simulink model "comparesansetavec"  (R2017a)
settings: Solver=VariableStepAuto  StartTime=0.0  StopTime=30  RelTol=1e-3
settings Model: Creator=pc  LastModifiedBy=pc

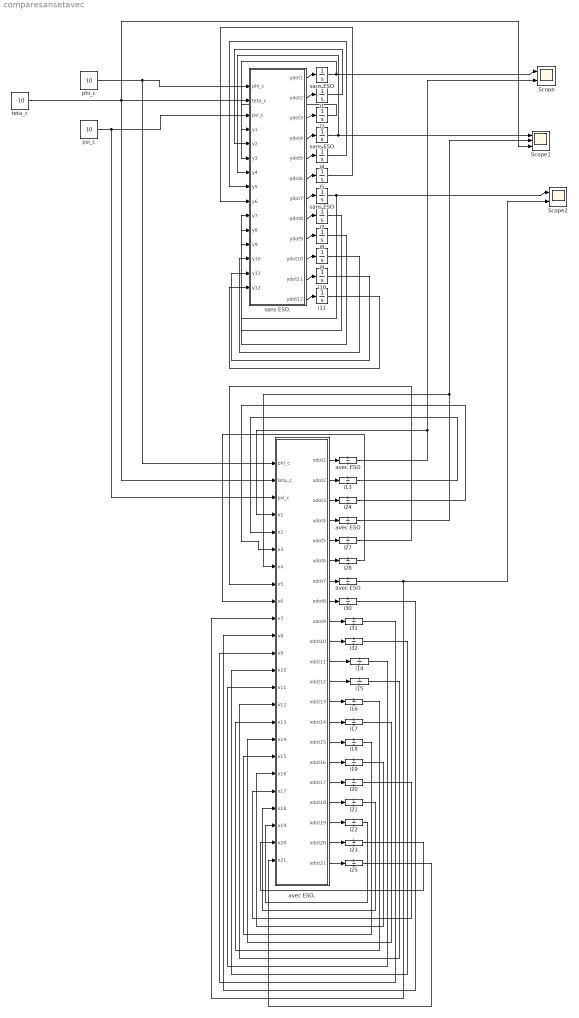
== system comparesansetavec ==
  Scope : Scope  NumInputPorts=2
  Scope1 : Scope  NumInputPorts=3
  Scope2 : Scope  NumInputPorts=2
  avec ESO : Integrator
  "avec ESO " : Integrator
  "avec ESO  " : Integrator
  avec ESO. : MATLAB Function  TreatAsAtomicUnit=on
  i{1..2,4..5,7..11,13..25,27..28,30..32} (27 alike) : Integrator
  phi_c : Constant  Value=10
  psi_c : Constant  Value=10
  sans ESO : Integrator
  "sans ESO " : Integrator
  "sans ESO  " : Integrator
  sans ESO. : MATLAB Function  TreatAsAtomicUnit=on
  teta_c : Constant  Value=-10
  wires:
  i10/1 -> sans ESO./14(y11)
  i5/1 -> sans ESO./9(y6)
  i7/1 -> sans ESO./11(y8)
  i1/1 -> sans ESO./5(y2)
  sans ESO./7(ydot7) -> "sans ESO "/1
  i2/1 -> sans ESO./6(y3)
  "sans ESO "/1 -> Scope2/1, sans ESO./10(y7)
  "sans ESO  "/1 -> Scope/1, sans ESO./4(y1)
  sans ESO./10(ydot10) -> i9/1
  sans ESO./4(ydot4) -> sans ESO/1
  sans ESO./3(ydot3) -> i2/1
  sans ESO/1 -> Scope1/1, sans ESO./7(y4)
  i4/1 -> sans ESO./8(y5)
  sans ESO./2(ydot2) -> i1/1
  sans ESO./9(ydot9) -> i8/1
  i11/1 -> sans ESO./15(y12)
  sans ESO./12(ydot12) -> i11/1
  sans ESO./1(ydot1) -> "sans ESO  "/1
  sans ESO./8(ydot8) -> i7/1
  sans ESO./11(ydot11) -> i10/1
  i8/1 -> sans ESO./12(y9)
  sans ESO./6(ydot6) -> i5/1
  i9/1 -> sans ESO./13(y10)
  sans ESO./5(ydot5) -> i4/1
  avec ESO./6(xdot6) -> i28/1
  i28/1 -> avec ESO./9(x6)
  i13/1 -> avec ESO./5(x2)
  avec ESO./14(xdot14) -> i17/1
  i17/1 -> avec ESO./17(x14)
  avec ESO./13(xdot13) -> i16/1
  avec ESO./2(xdot2) -> i13/1
  i22/1 -> avec ESO./22(x19)
  avec ESO./5(xdot5) -> i27/1
  avec ESO./9(xdot9) -> i31/1
  i25/1 -> avec ESO./24(x21)
  i21/1 -> avec ESO./21(x18)
  i20/1 -> avec ESO./20(x17)
  avec ESO./3(xdot3) -> i24/1
  avec ESO./12(xdot12) -> i15/1
  i15/1 -> avec ESO./15(x12)
  avec ESO./4(xdot4) -> avec ESO/1
  "avec ESO  "/1 -> Scope/2, avec ESO./4(x1)
  i23/1 -> avec ESO./23(x20)
  avec ESO/1 -> Scope1/2, avec ESO./7(x4)
  phi_c/1 -> avec ESO./1(phi_c), sans ESO./1(phi_c)
  i24/1 -> avec ESO./6(x3)
  i16/1 -> avec ESO./16(x13)
  "avec ESO "/1 -> avec ESO./10(x7), Scope2/2
  psi_c/1 -> avec ESO./3(psi_c), sans ESO./3(psi_c)
  i30/1 -> avec ESO./11(x8)
  i18/1 -> avec ESO./18(x15)
  teta_c/1 -> avec ESO./2(teta_c), Scope1/3, sans ESO./2(teta_c)
  avec ESO./18(xdot18) -> i21/1
  i27/1 -> avec ESO./8(x5)
  i31/1 -> avec ESO./12(x9)
  avec ESO./8(xdot8) -> i30/1
  avec ESO./1(xdot1) -> "avec ESO  "/1
  avec ESO./10(xdot10) -> i32/1
  avec ESO./16(xdot16) -> i19/1
  avec ESO./15(xdot15) -> i18/1
  avec ESO./21(xdot21) -> i25/1
  avec ESO./19(xdot19) -> i22/1
  avec ESO./7(xdot7) -> "avec ESO "/1
  avec ESO./20(xdot20) -> i23/1
  i19/1 -> avec ESO./19(x16)
  i14/1 -> avec ESO./14(x11)
  avec ESO./11(xdot11) -> i14/1
  i32/1 -> avec ESO./13(x10)
  avec ESO./17(xdot17) -> i20/1

== matlab function comparesansetavec/avec ESO. ==
  data: phi_c input; teta_c input; psi_c input; xdot1 output; x1 input; x2 input; x3 input; x4 input; x5 input; x6 input; x7 input; x8 input; x9 input; x10 input; x11 input; x12 input; x13 input; x14 input; x15 input; x16 input; x17 input; x18 input; x19 input; x20 input; x21 input; xdot2 output; xdot3 output; xdot4 output; xdot5 output; xdot6 output; xdot7 output; xdot8 output; xdot9 output; xdot10 output; xdot11 output; xdot12 output; xdot13 output; xdot14 output; xdot15 output; xdot16 output; xdot17 output; xdot18 output; xdot19 output; xdot20 output; xdot21 output
function [xdot1,xdot2,xdot3,xdot4,xdot5,xdot6,xdot7,xdot8,xdot9,xdot10,xdot11,xdot12,xdot13,xdot14,xdot15,xdot16,xdot17,xdot18,xdot19,xdot20,xdot21] = fcn(phi_c,teta_c,psi_c,x1,x2,x3,x4,x5,x6,x7,x8,x9,x10,x11,x12,x13,x14,x15,x16,x17,x18,x19,x20,x21)
alfa1=0.9; alfa2=0.3;
delta=0.1;
kd1=6.4;kd2=6.4;kd3=6.4;
kp1=16;kp2=16;kp3=16;
beta1=100; beta2=3000; beta3=5000;
%--------------------------------------------------------------------------
Ix=22682;
Iy=77095;
Iz=95561;
Ixz=1125;
SOM=Ix*Iz-Ixz^2;
c1=((Iy-Iz)*Iz-Ixz^2)/SOM;
c2=((Ix-Iy+Iz)*Ixz)/SOM;
c3=Iz/SOM;
c4=Ixz/SOM;
c5=(Iz-Ix)/Iy;
c6=Ixz/Iy;
c7=1/Iy;
c8=(Ix*(Ix-Iy)+Ixz^2)/SOM;
c9=Ix/SOM;
%--------------------------------------------------------------------------
phi=x1;
teta=x4;
p=x19;
r=x20;
q=x21;
%--------------------------------------------------------------------------
B=[c3+c4*cosd(phi)*tand(teta),c7*sind(phi)*tand(teta),c4+c9*cosd(phi)*tand(teta);
    -c4*sind(phi),c7*cosd(phi),-c9*sind(phi);
    c4*cosd(phi)*(1/cosd(teta)),c7*sind(phi)*(1/cosd(teta)),c9*cosd(phi)*(1/cosd(teta))];
phidot=p+tand(teta)*(q*sind(phi)+r*cosd(phi));
tetadot=q*cosd(phi)-r*sind(phi);
A1=((c1*r+c2*p)*q)+(tetadot/cosd(teta)^2)*(q*sind(phi)+r*cosd(phi))+tand(teta)*((c5*p*r-c6*(p^2-r^2))*sind(phi)+q*(phidot*cosd(phi))+((c8*p-c2*r)*q)*cosd(phi)-r*phidot*sind(phi));
A2=(c5*p*r-c6*(p^2-r^2))*cosd(phi)-phidot*sind(phi)*q-(((c8*p-c2*r)*q)*sind(phi)+phidot*cosd(phi)*r);
A3=((c5*p*r-c6*(p^2-r^2))*sind(phi)+phidot*cosd(phi)*q+((c8*p-c2*r)*q)*cosd(phi)-phidot*sind(phi)*r)*cosd(teta)/cosd(teta)^2+(tetadot*sind(teta)*(q*sind(phi)+r*cosd(phi)))/cosd(teta)^2;
%--------------------------------------------------------------------------
pp=inv(B);
L=pp(1,:)*[(kp1*phi_c-x12)-A1;(kp2*teta_c-x15)-A2;(kp3*psi_c-x18)-A3];
M=pp(2,:)*[(kp1*phi_c-x12)-A1;(kp2*teta_c-x15)-A2;(kp3*psi_c-x18)-A3];
N=pp(3,:)*[(kp1*phi_c-x12)-A1;(kp2*teta_c-x15)-A2;(kp3*psi_c-x18)-A3];
%************------************----------**************-----------------
e=x10-x1;                                     %y(1)=phi y(10)=Z1_phi 
e2=x13-x4;                                      %y(4)=teta y(14)=Z1_teta
e3=x16-x7;                                      %y(7)=psi y(16)=Z1_PSI
%************------************----------**************-----------------
xdot1=x2;   
%xdot2=A1+B(1,:)*[L;M;N];
xdot2=x3+kp1*phi_c;
%xdot3=A1dot+Bdot(1,:)*u+B(1,:)*udot;
Delta_u1=x12+kp1*x1+kd1*x2;
xdot3=-kp1*x2-kd1*(x3+kp1*phi_c)-Delta_u1;
%---ESO1 Z_PHI---
xdot10=x11-beta1*e;                           %y(11)=Z2_phi
%^^^^^^^^^^^^^^^^^^^^^^^^^^^^^^^^^^^^^^^^^^^^^^^^^^^^^^^^^^^^^^^^^^^^^^^^^^
if abs(e)> delta 
FAL=abs(e)^alfa1*sign(e);
xdot11=x12-beta2*FAL+kp1*phi_c;%y(12)=Z3_phi
else 
    FAL=e/(delta^(1-alfa1));
 xdot11=x12-beta2*FAL+kp1*phi_c;%y(12)=Z3_phi
end
%^^^^^^^^^^^^^^^^^^^^^^^^^^^^^^^^^^^^^^^^^^^^^^^^^^^^^^^^^^^^^^^^^^^^^^^^^^ 
if abs(e)> delta 
FAL1=abs(e)^alfa2*sign(e);
xdot12=-beta3*FAL1;
else 
    FAL1=e/(delta^(1-alfa2));
    xdot12=-beta3*FAL1;
end
%^^^^^^^^^^^^^^^^^^^^^^^^^^^^^^^^^^^^^^^^^^^^^^^^^^^^^^^^^^^^^^^^^^^^^^^^^^


%--------------------------------------------------------------------------
xdot4=x5;   
%xdot4=A2+B(2,:)*[L;M;N];  
xdot5=x6+kp2*teta_c;
%xdot6=A2dot+Bdot(2,:)*u+B(2,:)*udot;
Delta_u2=x15+kp2*x4+kd2*x5;
xdot6=-kp2*x5-kd1*(x6+kp2*teta_c)-Delta_u2;
%---ESO2 Z_Teta---
xdot13=x14-beta1*e2;                            %y(15)=Z2_teta
%^^^^^^^^^^^^^^^^^^^^^^^^^^^^^^^^^^^^^^^^^^^^^^^^^^^^^^^^^^^^^^^^^^^^^^^^^^
if abs(e2)> delta 
FAL2=abs(e2)^alfa1*sign(e2);
xdot14=x15-beta2*FAL2+kp2*teta_c;%y(16)=Z3_teta 
else
    FAL2=e2/(delta^(1-alfa1));
xdot14=x15-beta2*FAL2+kp2*teta_c;%y(16)=Z3_teta 
end
%^^^^^^^^^^^^^^^^^^^^^^^^^^^^^^^^^^^^^^^^^^^^^^^^^^^^^^^^^^^^^^^^^^^^^^^^^^ 
if abs(e2)> delta 
FAL3=abs(e2)^alfa2*sign(e2);
xdot15=-beta3*FAL3;
else
    FAL3=e2/(delta^(1-alfa2));
xdot15=-beta3*FAL3;
end
%^^^^^^^^^^^^^^^^^^^^^^^^^^^^^^^^^^^^^^^^^^^^^^^^^^^^^^^^^^^^^^^^^^^^^^^^^^


%--------------------------------------------------------------------------
xdot7=x8;   
%xdot6=A3+B(3,:)*[L;M;N];
xdot8=x9+kp3*psi_c;
%xdot9=A3dot+Bdot(3,:)*u+B(3,:)*udot;
Delta_u3=x18+kp3*x7+kd3*x8;
xdot9=-kp3*x8-kd3*(x9+kp3*psi_c)-Delta_u3;
%---ESO3 Z_PSI---
xdot16=x17-beta1*e3;                          %y(17)=Z2_PSI
%^^^^^^^^^^^^^^^^^^^^^^^^^^^^^^^^^^^^^^^^^^^^^^^^^^^^^^^^^^^^^^^^^^^^^^^^^^
if abs(e3)> delta 
FAL4=abs(e3)^alfa1*sign(e3);
xdot17=x18-beta2*FAL4+kp3*psi_c; %y(18)=Z3_PSI
else
    FAL4=e3/(delta^(1-alfa1));
xdot17=x18-beta2*FAL4+kp3*psi_c; %y(18)=Z3_PSI
end
%^^^^^^^^^^^^^^^^^^^^^^^^^^^^^^^^^^^^^^^^^^^^^^^^^^^^^^^^^^^^^^^^^^^^^^^^^^ 
if abs(e3)> delta 
FAL5=abs(e3)^alfa2*sign(e3);
xdot18=-beta3*FAL5;
else
    FAL5=e3/(delta^(1-alfa2));
xdot18=-beta3*FAL5;
end
%^^^^^^^^^^^^^^^^^^^^^^^^^^^^^^^^^^^^^^^^^^^^^^^^^^^^^^^^^^^^^^^^^^^^^^^^^^

%--------------------------------------------------------------------------
xdot19=(c1*r+c2*p)*q+c3*L+c4*N;  %=pdot
xdot20=(c8*p-c2*r)*q+c4*L+c9*N;  %=rdot
xdot21=c5*p*r-c6*(p^2-r^2)+c7*M; %=qdot
end

== matlab function comparesansetavec/sans ESO. ==
  data: phi_c input; teta_c input; psi_c input; y1 input; ydot1 output; y2 input; y3 input; y4 input; y5 input; y6 input; y7 input; y8 input; y9 input; y10 input; y11 input; y12 input; ydot2 output; ydot3 output; ydot4 output; ydot5 output; ydot6 output; ydot7 output; ydot8 output; ydot9 output; ydot10 output; ydot11 output; ydot12 output
function [ydot1,ydot2,ydot3,ydot4,ydot5,ydot6,ydot7,ydot8,ydot9,ydot10,ydot11,ydot12] = fcn(phi_c,teta_c,psi_c,y1,y2,y3,y4,y5,y6,y7,y8,y9,y10,y11,y12)
kd1=6.4;kd2=6.4;kd3=6.4;
kp1=16;kp2=16;kp3=16;
%--------------------------------------------------------------------------
% Ix=12874.8;
% Iy=75673.6;
% Iz=85552.1;
% Ixz=1331.4;
Ix=22682;
Iy=77095;
Iz=95561;
Ixz=1125;
SOM=Ix*Iz-Ixz^2;
c1=((Iy-Iz)*Iz-Ixz^2)/SOM;
c2=((Ix-Iy+Iz)*Ixz)/SOM;
c3=Iz/SOM;
c4=Ixz/SOM;
c5=(Iz-Ix)/Iy;
c6=Ixz/Iy;
c7=1/Iy;
c8=(Ix*(Ix-Iy)+Ixz^2)/SOM;
c9=Ix/SOM;
%--------------------------------------------------------------------------
phi=y1;
teta=y4;
p=y10;
r=y11;
q=y12;
%--------------------------------------------------------------------------
B=[c3+c4*cosd(phi)*tand(teta),c7*sind(phi)*tand(teta),c4+c9*cosd(phi)*tand(teta);
    -c4*sind(phi),c7*cosd(phi),-c9*sind(phi);
    c4*cosd(phi)*(1/cosd(teta)),c7*sind(phi)*(1/cosd(teta)),c9*cosd(phi)*(1/cosd(teta))];
phidot=p+tand(teta)*(q*sind(phi)+r*cosd(phi));
tetadot=q*cosd(phi)-r*sind(phi);
A1=((c1*r+c2*p)*q)+(tetadot/cosd(teta)^2)*(q*sind(phi)+r*cosd(phi))+tand(teta)*((c5*p*r-c6*(p^2-r^2))*sind(phi)+q*(phidot*cosd(phi))+((c8*p-c2*r)*q)*cosd(phi)-r*phidot*sind(phi));
A2=(c5*p*r-c6*(p^2-r^2))*cosd(phi)-phidot*sind(phi)*q-(((c8*p-c2*r)*q)*sind(phi)+phidot*cosd(phi)*r);
A3=((c5*p*r-c6*(p^2-r^2))*sind(phi)+phidot*cosd(phi)*q+((c8*p-c2*r)*q)*cosd(phi)-phidot*sind(phi)*r)*cosd(teta)/cosd(teta)^2+(tetadot*sind(teta)*(q*sind(phi)+r*cosd(phi)))/cosd(teta)^2;
A=[A1;A2;A3];
%--------------------------------------------------------------------------
Bdot=[c4*cosd(phi)*(tand(teta)^2 + 1)*tetadot - c4*sind(phi)*tand(teta)*phidot,c7*cosd(phi)*tand(teta)*phidot + c7*sind(phi)*(tand(teta)^2 + 1)*tetadot,c9*cosd(phi)*(tand(teta)^2 + 1)*tetadot - c9*sind(phi)*tand(teta)*phidot;
     -c4*cosd(phi)*phidot,-c7*sind(phi)*phidot,-c9*cosd(phi)*phidot;
     (c4*cosd(phi)*sind(teta)*tetadot)/cosd(teta)^2 - (c4*sind(phi)*phidot)/cosd(teta), (c7*cosd(phi)*phidot)/cosd(teta) + (c7*sind(phi)*sind(teta)*tetadot)/cosd(teta)^2, (c9*cosd(phi)*sind(teta)*tetadot)/cosd(teta)^2 - (c9*sind(phi)*phidot)/cosd(teta)];
%--------------------------------------------------------------------------
pp=inv(B);
L=pp(1,:)*[(kp1*(phi_c-y1)-kd1*y2)-A1;((kp2*(teta_c-y4)-kd2*y5)-A2);((kp3*(psi_c-y7)-kd3*y8)-A3)];
M=pp(2,:)*[(kp1*(phi_c-y1)-kd1*y2)-A1;((kp2*(teta_c-y4)-kd2*y5)-A2);((kp3*(psi_c-y7)-kd3*y8)-A3)];
N=pp(3,:)*[(kp1*(phi_c-y1)-kd1*y2)-A1;((kp2*(teta_c-y4)-kd2*y5)-A2);((kp3*(psi_c-y7)-kd3*y8)-A3)];
pdot=(c1*r+c2*p)*q+c3*L+c4*N;
rdot=(c8*p-c2*r)*q+c4*L+c9*N;
qdot=c5*p*r-c6*(p^2-r^2)+c7*M;

phidotdot=pdot+(tetadot/cosd(teta)^2)*(q*sind(phi)+r*cosd(phi))+tand(teta)*(qdot*sind(phi)+q*(phidot*cosd(phi))+rdot*cosd(phi)-r*phidot*sind(phi));
tetadotdot=qdot*cosd(phi)-phidot*sind(phi)*q-(rdot*sind(phi)+phidot*cosd(phi)*r);

A1dot=(c1*rdot+c2*pdot)*q+qdot*(c1*r+c2*p)+(tetadotdot*cosd(teta)^2+2*tetadot^2*sind(teta)*cosd(teta))/cosd(teta)^4*(q*sind(phi)+r*cosd(phi))+(qdot*sind(phi)+phidot*cosd(phi)*q+rdot*cosd(phi)-phidot*sind(phi)*r)*(tetadot/cosd(teta)^2)+(tetadot/cosd(teta)^2)*((c5*p*r-c6*(p^2-r^2))*sind(phi)+q*(phidot*cosd(phi))+((c8*p-c2*r)*q)*cosd(phi)-r*phidot*sind(phi))+((c5*p*r-c6*(p^2-r^2))*phidot*cosd(phi)+(c5*(pdot*r+rdot*p)-c6*(2*p*pdot-2*r*rdot))*sind(phi)+(qdot*phidot+phidotdot*q)*cosd(phi)-phidot*sind(phi)*q*phidot+(c8*pdot-c2*rdot)*q*cosd(phi)+(qdot*cosd(phi)-phidot*sind(phi)*q)*(c8*p-c2*r)-((rdot*phidot+phidotdot*r)*sind(phi)+phidot*cosd(phi)*r*phidot))*tand(teta);
A2dot=(c5*(pdot*r+rdot*p)-c6*(2*p*pdot-2*r*rdot))*cosd(phi)-phidot*sind(phi)*(c5*p*r-c6*(p^2-r^2))-((phidotdot*q+qdot*phidot)*sind(phi)+phidot*cosd(phi)*phidot*q)-(((c8*pdot-c2*rdot)*q+qdot*(c8*p-c2*r))*sind(phi)+phidot*cosd(phi)*((c8*p-c2*r)*q)+(phidotdot*r+rdot*phidot)*cosd(phi)-phidot*sind(phi)*phidot*r);
A3dot=((((c5*(pdot*r+rdot*p)-c6*(2*p*pdot-2*r*rdot))*sind(phi)+phidot*cosd(phi)*(c5*p*r-c6*(p^2-r^2))+(phidotdot*cosd(phi)-phidot*sind(phi)*phidot)*q+qdot*phidot*cosd(phi)+((c8*pdot-c2*rdot)*q+qdot*(c8*p-c2*r))*cosd(phi)-phidot*sind(phi)*((c8*p-c2*r)*q)-((phidotdot*sind(phi)+phidot*cosd(phi)*phidot)*r+rdot*phidot*sind(phi)))*cosd(teta)-tetadot*sind(teta)*((c5*p*r-c6*(p^2-r^2))*sind(phi)+phidot*cosd(phi)*q+(c5*p*r-c6*(p^2-r^2))*cosd(phi)-phidot*sind(phi)*r))*cosd(teta)^2+2*tetadot*cosd(teta)*sind(teta)*((c5*p*r-c6*(p^2-r^2))*sind(phi)+phidot*cosd(phi)*q+((c8*p-c2*r)*q)*cosd(phi)-phidot*sind(phi)*r)*cosd(teta))/cosd(teta)^4+(((tetadotdot*sind(teta)+tetadot*cosd(teta)*tetadot)*(q*sind(phi)+r*cosd(phi))+(qdot*sind(phi)+phidot*cosd(phi)*q+rdot*cosd(phi)-phidot*sind(phi)*r)*tetadot*sind(teta))*cosd(teta)^2+2*tetadot*cosd(teta)*sind(teta)*(tetadot*sind(teta)*(q*sind(phi)+r*cosd(phi))))/cosd(teta)^4;
Adot=[A1dot;A2dot;A3dot];
%--------------------------------------------------------------------------
u=[L;M;N];
ppdot=[ 0, -(c4*cosd(phi)*phidot)/(c4^2*cosd(phi)^2 + c4^2*sind(phi)^2 - c3*c9*cosd(phi)^2 - c3*c9*sind(phi)^2), (cosd(teta)*(c9*cosd(phi)^2*(tand(teta)^2 + 1)*tetadot - c4*sind(phi)*phidot + c9*sind(phi)^2*(tand(teta)^2 + 1)*tetadot))/(c4^2*cosd(phi)^2 + c4^2*sind(phi)^2 - c3*c9*cosd(phi)^2 - c3*c9*sind(phi)^2) - (sind(teta)*tetadot*(c9*tand(teta)*cosd(phi)^2 + c4*cosd(phi) + c9*tand(teta)*sind(phi)^2))/(c4^2*cosd(phi)^2 + c4^2*sind(phi)^2 - c3*c9*cosd(phi)^2 - c3*c9*sind(phi)^2);
        0,                                                    -(sind(phi)*phidot)/(c7*cosd(phi)^2 + c7*sind(phi)^2),                                                                                                                                                                                                                                                                                             (cosd(phi)*cosd(teta)*phidot)/(c7*cosd(phi)^2 + c7*sind(phi)^2) - (sind(phi)*sind(teta)*tetadot)/(c7*cosd(phi)^2 + c7*sind(phi)^2);
        0,  (c3*cosd(phi)*phidot)/(c4^2*cosd(phi)^2 + c4^2*sind(phi)^2 - c3*c9*cosd(phi)^2 - c3*c9*sind(phi)^2), (sind(teta)*tetadot*(c4*tand(teta)*cosd(phi)^2 + c3*cosd(phi) + c4*tand(teta)*sind(phi)^2))/(c4^2*cosd(phi)^2 + c4^2*sind(phi)^2 - c3*c9*cosd(phi)^2 - c3*c9*sind(phi)^2) - (cosd(teta)*(c4*cosd(phi)^2*(tand(teta)^2 + 1)*tetadot - c3*sind(phi)*phidot + c4*sind(phi)^2*(tand(teta)^2 + 1)*tetadot))/(c4^2*cosd(phi)^2 + c4^2*sind(phi)^2 - c3*c9*cosd(phi)^2 - c3*c9*sind(phi)^2)];
v=[(kp1*(phi_c-y1)-kd1*y2);(kp2*(teta_c-y4)-kd2*y5);(kp3*(psi_c-y7)-kd3*y8)];
vdot=[-kp1*y2-kd1*(y3+kp1*phi_c);-kp2*y5-kd2*(y6+kp2*teta_c);-kp3*y8-kd3*(y9+kp3*psi_c)];
udot=ppdot*(v-A)+pp*(vdot-Adot);
%--------------------------------------------------------------------------
ydot1=y2;   
%ydot(2)=A1+B(1,:)*[L;M;N];
ydot2=y3+kp1*phi_c;
ydot3=A1dot+Bdot(1,:)*u+B(1,:)*udot;
%--------------------------------------------------------------------------
ydot4=y5;   
%ydot(4)=A2+B(2,:)*[L;M;N];  
ydot5=y6+kp2*teta_c;
ydot6=A2dot+Bdot(2,:)*u+B(2,:)*udot;
%--------------------------------------------------------------------------
ydot7=y8;   
%ydot(6)=A3+B(3,:)*[L;M;N];
ydot8=y9+kp3*psi_c;
ydot9=A3dot+Bdot(3,:)*u+B(3,:)*udot;
%--------------------------------------------------------------------------
ydot10=(c1*r+c2*p)*q+c3*L+c4*N;  %=pdot
ydot11=(c8*p-c2*r)*q+c4*L+c9*N;  %=rdot
ydot12=c5*p*r-c6*(p^2-r^2)+c7*M; %=qdot
end
